simulink model "tsl235rtest"  (R2013b)
settings: Solver=ode45  StartTime=0.0  StopTime=5  RelTol=1e-3
libraries: simulink x2
settings Model: Creator=Markus  LastModifiedBy=Markus

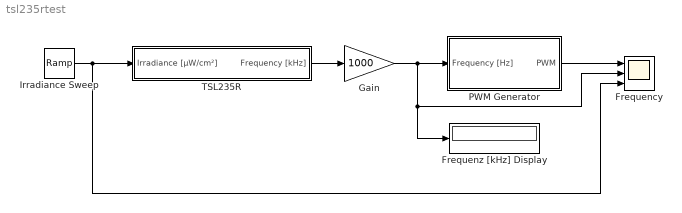
== system tsl235rtest ==
  Frequency : Scope  NumInputPorts=3
      settings: YMin=-5~-5~-5  YMax=5~5~5
  Frequenz [kHz] Display : Display
  Gain : Gain  Gain=1000
  Irradiance Sweep : simulink/Sources/Ramp  slope=0.01  start=0  X0=0
  PWM Generator : Subsystem
  TSL235R : Subsystem
  wires:
  Irradiance Sweep/1 -> Frequency/3, TSL235R/1(Irradiance [µW/cm²])
  TSL235R/1(Frequency [kHz]) -> Gain/1
  Gain/1 -> PWM Generator/1(Frequency [Hz]), Frequenz [kHz] Display/1, Frequency/2
  PWM Generator/1(PWM) -> Frequency/1

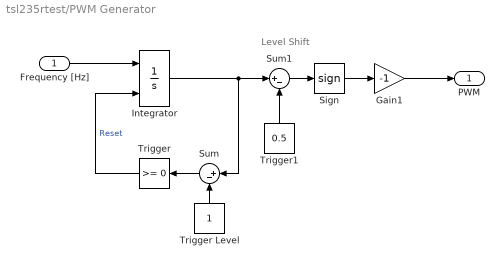
== system tsl235rtest/PWM Generator ==
  note: Level Shift
  Frequency [Hz] : Inport
  Gain1 : Gain  Gain=-1
  Integrator : Integrator  ExternalReset=rising
  Sign : Signum
  Sum : Sum  Inputs=|+-
  Sum1 : Sum  Inputs=|+-
  Trigger : simulink/Logic and Bit Operations/Compare To Zero  relop=>=  OutDataTypeStr=boolean
  Trigger Level : Constant
  Trigger1 : Constant  Value=0.5
  PWM : Outport
  wires:
  Trigger/1 -> Integrator/2  "Reset"
  Sum/1 -> Trigger/1
  Sum1/1 -> Sign/1
  Trigger Level/1 -> Sum/2
  Integrator/1 -> Sum1/1, Sum/1
  Gain1/1 -> PWM/1
  Frequency [Hz]/1 -> Integrator/1
  Sign/1 -> Gain1/1
  Trigger1/1 -> Sum1/2

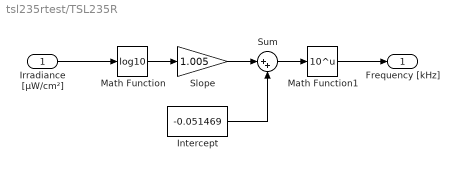
== system tsl235rtest/TSL235R ==
  Irradiance [µW/cm²] : Inport
  Intercept : Constant  Value=-0.051469
  Math Function : Math  Operator=log10  SaturateOnIntegerOverflow=on
  Math Function1 : Math  Operator=10^u  SaturateOnIntegerOverflow=on
  Slope : Gain  Gain=1.005
  Sum : Sum  Inputs=|++
  Frequency [kHz] : Outport
  wires:
  Irradiance [µW/cm²]/1 -> Math Function/1
  Slope/1 -> Sum/1
  Intercept/1 -> Sum/2
  Sum/1 -> Math Function1/1
  Math Function/1 -> Slope/1
  Math Function1/1 -> Frequency [kHz]/1
